simulink model "TAL8"  (Simulink 6.1)
settings: Solver=ode45  StartTime=0.0  StopTime=1000.0  RelTol=1e-3
values from neighbouring files (symbols this model uses):
  apr = 4    [data_TAL.m]
  apt = .3    (= 0.3)    [data_TAL.m]
  c_tal = 1    [data_TAL.m]
  egpith = -85    [data_synapses.m]
  ek_tal = -90    [data_TAL.m]
  el_tal = -70    [data_TAL.m]
  ena_tal = 50    [data_TAL.m]
  et_tal = 0    [data_TAL.m]
  ggpith = ggpith*mod_gpital    [CN_launch_CN_analyze_TAL2.m]    (also in CN_launch_sysTAL.m = ggpith*2; data_synapses.m = 0.06)
  gk_tal = 5    [data_TAL.m]
  gl_tal = 0.05    [data_TAL.m]
  gna_tal = 3    [data_TAL.m]
  gt_tal = 5    [data_TAL.m]
  ht0 = [i_v_16(322),i_v_16(325),i_v_16(322),i_v_16(325),i_v_16(322),i_v_16(325)]    [CN_launch_CN_analyze_TAL2.m]    (also in CN_launch_sysTAL.m)
  qht = 5.5    [data_TAL.m]
  rt0 = [i_v_16(323),i_v_16(326),i_v_16(323),i_v_16(326),i_v_16(323),i_v_16(326)]    [CN_launch_CN_analyze_TAL2.m]    (also in CN_launch_sysTAL.m)
  tadj = 1    [data_TAL.m]
  vt0 = [i_v_16(321),i_v_16(324),i_v_16(321),i_v_16(324),i_v_16(321),i_v_16(324)]    [CN_launch_CN_analyze_TAL2.m]    (also in CN_launch_sysTAL.m)
settings Model: LastModifiedBy=marco
settings DataIOCC: ExternalInput=[t2, u2]  LoadExternalInput=on
settings OptimizationCC: InlineInvariantSignals=off
settings DebuggingCC: SolverPrmCheckMsg=warning

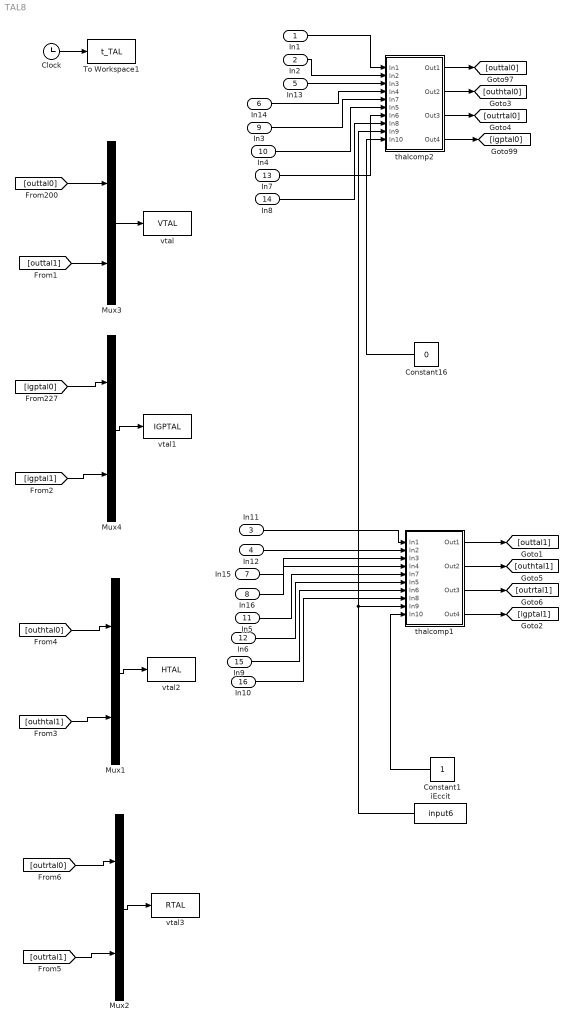
== system TAL8 ==
  In1 : Inport  Port=1  LatchInput=off
  In2 : Inport  Port=2  LatchInput=off
  In11 : Inport  Port=3  LatchInput=off
  In12 : Inport  Port=4  LatchInput=off
  In13 : Inport  Port=5  LatchInput=off
  In14 : Inport  Port=6  LatchInput=off
  In15 : Inport  Port=7  LatchInput=off
  In16 : Inport  Port=8  LatchInput=off
  In3 : Inport  Port=9  LatchInput=off
  In4 : Inport  Port=10  LatchInput=off
  In5 : Inport  Port=11  LatchInput=off
  In6 : Inport  Port=12  LatchInput=off
  In7 : Inport  Port=13  LatchInput=off
  In8 : Inport  Port=14  LatchInput=off
  In9 : Inport  Port=15  LatchInput=off
  In10 : Inport  Port=16  LatchInput=off
  Clock : Clock
      settings: Decimation=10
  Constant1 : Constant  Orientation=left
  Constant16 : Constant  Orientation=left  Value=0
  Mux{1..4} (4 alike) : Mux  Inputs=2
  To Workspace1 : ToWorkspace  VariableName=t_TAL  SampleTime=-1  SaveFormat=Array
  iEccit : FromWorkspace  Orientation=left  VariableName=input6  SampleTime=1
  thalcomp1 : Subsystem
  thalcomp2 : Subsystem
  vtal : ToWorkspace  VariableName=VTAL  SampleTime=-1  SaveFormat=Array
  vtal1 : ToWorkspace  VariableName=IGPTAL  SampleTime=-1  SaveFormat=Array
  vtal2 : ToWorkspace  VariableName=HTAL  SampleTime=-1  SaveFormat=Array
  vtal3 : ToWorkspace  VariableName=RTAL  SampleTime=-1  SaveFormat=Array
  wires:
  Clock/1 -> To Workspace1/1
  thalcomp2/1(Out1) -> [outtal0]
  In2/1 -> thalcomp2/2(In2)
  thalcomp2/4(Out4) -> [igptal0]
  In1/1 -> thalcomp2/1(In1)
  Mux3/1 -> vtal/1
  [outtal0] -> Mux3/1
  Mux4/1 -> vtal1/1
  [igptal0] -> Mux4/1
  In13/1 -> thalcomp2/3(In3)
  In14/1 -> thalcomp2/4(In4)
  Constant16/1 -> thalcomp2/10(In10)
  iEccit/1 -> thalcomp2/9(In9), thalcomp1/9(In9)
  In3/1 -> thalcomp2/5(In7)
  In4/1 -> thalcomp2/6(In5)
  In7/1 -> thalcomp2/7(In6)
  In8/1 -> thalcomp2/8(In8)
  Constant1/1 -> thalcomp1/10(In10)
  In11/1 -> thalcomp1/1(In1)
  In12/1 -> thalcomp1/2(In2)
  In15/1 -> thalcomp1/3(In3)
  In16/1 -> thalcomp1/4(In4)
  In5/1 -> thalcomp1/5(In7)
  In6/1 -> thalcomp1/6(In5)
  In9/1 -> thalcomp1/7(In6)
  In10/1 -> thalcomp1/8(In8)
  thalcomp1/1(Out1) -> [outtal1]
  thalcomp1/4(Out4) -> [igptal1]
  [outtal1] -> Mux3/2
  [igptal1] -> Mux4/2
  thalcomp2/2(Out2) -> [outhtal0]
  thalcomp2/3(Out3) -> [outrtal0]
  thalcomp1/2(Out2) -> [outhtal1]
  thalcomp1/3(Out3) -> [outrtal1]
  Mux1/1 -> vtal2/1
  [outhtal0] -> Mux1/1
  [outhtal1] -> Mux1/2
  Mux2/1 -> vtal3/1
  [outrtal0] -> Mux2/1
  [outrtal1] -> Mux2/2

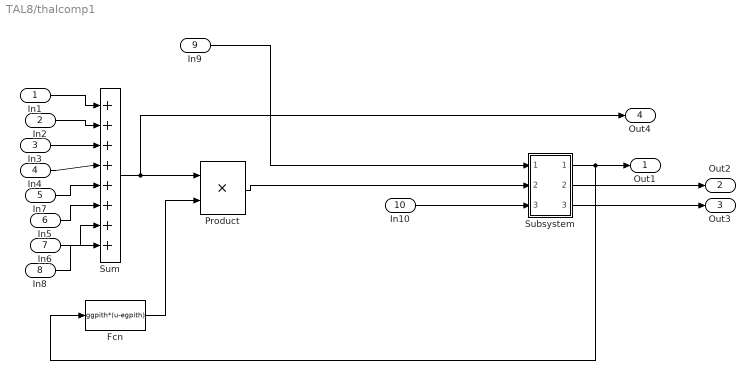
== system TAL8/thalcomp1 ==
  In1 : Inport  Port=1  LatchInput=off
  In2 : Inport  Port=2  LatchInput=off
  In3 : Inport  Port=3  LatchInput=off
  In4 : Inport  Port=4  LatchInput=off
  In7 : Inport  Port=5  LatchInput=off
  In5 : Inport  Port=6  LatchInput=off
  In6 : Inport  Port=7  LatchInput=off
  In8 : Inport  Port=8  LatchInput=off
  In9 : Inport  Port=9  LatchInput=off
  In10 : Inport  Port=10  LatchInput=off
  Fcn : Fcn  Expr=ggpith*(u-egpith)
  Product : Product  SaturateOnIntegerOverflow=on  InputSameDT=on
  Subsystem : Subsystem
  Sum : Sum  Inputs=++++++++  SaturateOnIntegerOverflow=on  InputSameDT=on
  Out1 : Outport
  Out2 : Outport  Port=2
  Out3 : Outport  Port=3
  Out4 : Outport  Port=4
  wires:
  Sum/1 -> Product/1, Out4/1
  Fcn/1 -> Product/2
  In1/1 -> Sum/1
  In2/1 -> Sum/2
  Product/1 -> Subsystem/2(In2)
  In9/1 -> Subsystem/1(In1)
  Subsystem/1(Out1) -> Fcn/1, Out1/1
  In10/1 -> Subsystem/3(In3)
  In4/1 -> Sum/4
  In3/1 -> Sum/3
  In8/1 -> Sum/8
  In6/1 -> Sum/7
  In5/1 -> Sum/6
  In7/1 -> Sum/5
  Subsystem/2(Out2) -> Out2/1
  Subsystem/3(Out3) -> Out3/1

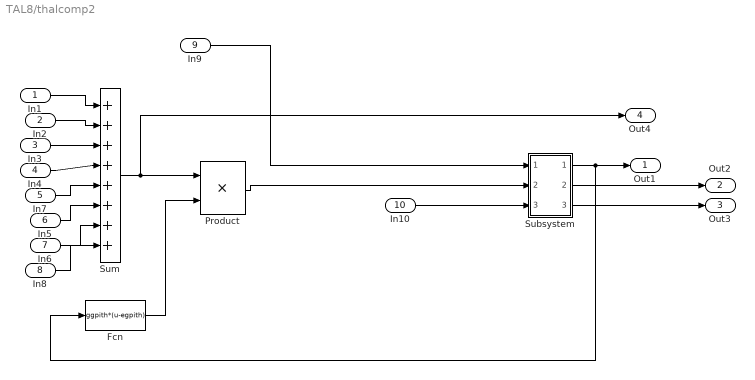
== system TAL8/thalcomp2 ==
  In1 : Inport  Port=1  LatchInput=off
  In2 : Inport  Port=2  LatchInput=off
  In3 : Inport  Port=3  LatchInput=off
  In4 : Inport  Port=4  LatchInput=off
  In7 : Inport  Port=5  LatchInput=off
  In5 : Inport  Port=6  LatchInput=off
  In6 : Inport  Port=7  LatchInput=off
  In8 : Inport  Port=8  LatchInput=off
  In9 : Inport  Port=9  LatchInput=off
  In10 : Inport  Port=10  LatchInput=off
  Fcn : Fcn  Expr=ggpith*(u-egpith)
  Product : Product  SaturateOnIntegerOverflow=on  InputSameDT=on
  Subsystem : Subsystem
  Sum : Sum  Inputs=++++++++  SaturateOnIntegerOverflow=on  InputSameDT=on
  Out1 : Outport
  Out2 : Outport  Port=2
  Out3 : Outport  Port=3
  Out4 : Outport  Port=4
  wires:
  Sum/1 -> Product/1, Out4/1
  Fcn/1 -> Product/2
  In1/1 -> Sum/1
  In2/1 -> Sum/2
  Product/1 -> Subsystem/2(In2)
  In9/1 -> Subsystem/1(In1)
  Subsystem/1(Out1) -> Fcn/1, Out1/1
  In10/1 -> Subsystem/3(In3)
  In4/1 -> Sum/4
  In3/1 -> Sum/3
  In8/1 -> Sum/8
  In6/1 -> Sum/7
  In5/1 -> Sum/6
  In7/1 -> Sum/5
  Subsystem/2(Out2) -> Out2/1
  Subsystem/3(Out3) -> Out3/1

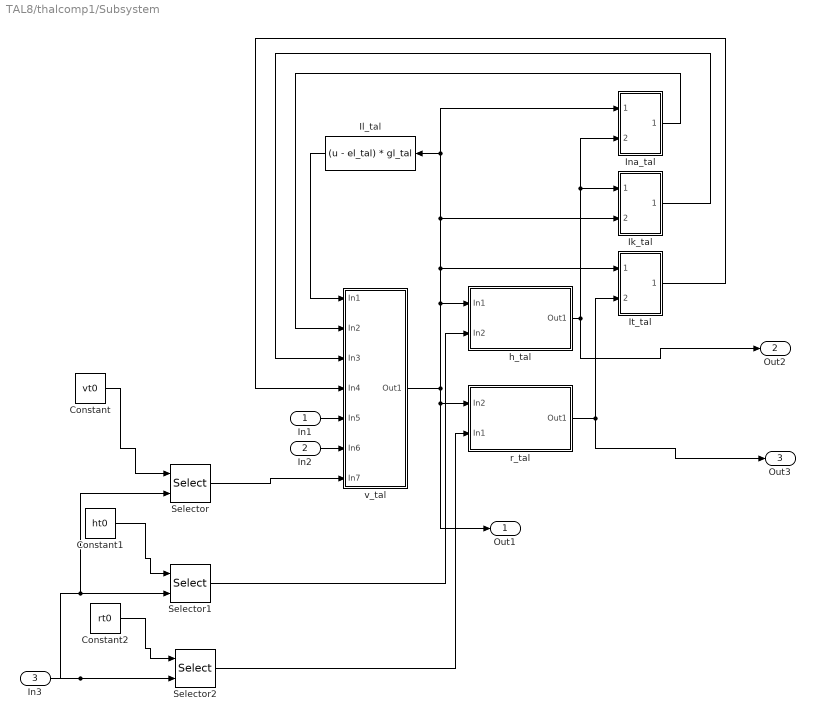
== system TAL8/thalcomp1/Subsystem ==
  In1 : Inport  Port=1  LatchInput=off
  In2 : Inport  Port=2  LatchInput=off
  In3 : Inport  Port=3  LatchInput=off
  Constant : Constant  Value=vt0
  Constant1 : Constant  Value=ht0
  Constant2 : Constant  Value=rt0
  Ik_tal : Subsystem
  Il_tal : Fcn  Orientation=left  Expr=(u - el_tal) * gl_tal
  Ina_tal : Subsystem
  It_tal : Subsystem
  Selector : Selector  IndexMode=Zero-based  ElementSrc=External  Elements=[1 3]
  Selector1 : Selector  IndexMode=Zero-based  ElementSrc=External  Elements=[1 3]
  Selector2 : Selector  IndexMode=Zero-based  ElementSrc=External  Elements=[1 3]
  h_tal : Subsystem
  r_tal : Subsystem
  v_tal : Subsystem
  Out1 : Outport
  Out2 : Outport  Port=2
  Out3 : Outport  Port=3
  wires:
  Il_tal/1 -> v_tal/1(In1)
  Ina_tal/1(Out1) -> v_tal/2(In2)
  Ik_tal/1(Out1) -> v_tal/3(In3)
  h_tal/1(Out1) -> Ik_tal/1(In1), Ina_tal/2(In2), Out2/1
  r_tal/1(Out1) -> It_tal/2(In2), Out3/1
  It_tal/1(Out1) -> v_tal/4(In4)
  v_tal/1(Out1) -> Il_tal/1, Ina_tal/1(In1), Ik_tal/2(In2), It_tal/1(In1), h_tal/1(In1), r_tal/1(In2), Out1/1
  In1/1 -> v_tal/5(In5)
  In2/1 -> v_tal/6(In6)
  In3/1 -> Selector2/2, Selector1/2, Selector/2
  Constant/1 -> Selector/1
  Selector/1 -> v_tal/7(In7)
  Constant1/1 -> Selector1/1
  Selector1/1 -> h_tal/2(In2)
  Constant2/1 -> Selector2/1
  Selector2/1 -> r_tal/2(In1)

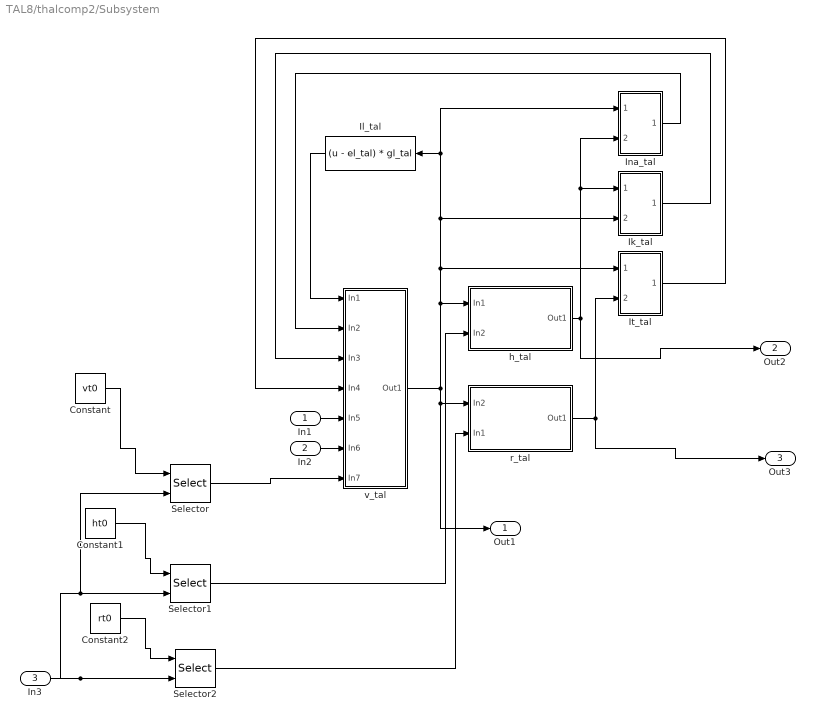
== system TAL8/thalcomp2/Subsystem ==
  In1 : Inport  Port=1  LatchInput=off
  In2 : Inport  Port=2  LatchInput=off
  In3 : Inport  Port=3  LatchInput=off
  Constant : Constant  Value=vt0
  Constant1 : Constant  Value=ht0
  Constant2 : Constant  Value=rt0
  Ik_tal : Subsystem
  Il_tal : Fcn  Orientation=left  Expr=(u - el_tal) * gl_tal
  Ina_tal : Subsystem
  It_tal : Subsystem
  Selector : Selector  IndexMode=Zero-based  ElementSrc=External  Elements=[1 3]
  Selector1 : Selector  IndexMode=Zero-based  ElementSrc=External  Elements=[1 3]
  Selector2 : Selector  IndexMode=Zero-based  ElementSrc=External  Elements=[1 3]
  h_tal : Subsystem
  r_tal : Subsystem
  v_tal : Subsystem
  Out1 : Outport
  Out2 : Outport  Port=2
  Out3 : Outport  Port=3
  wires:
  Il_tal/1 -> v_tal/1(In1)
  Ina_tal/1(Out1) -> v_tal/2(In2)
  Ik_tal/1(Out1) -> v_tal/3(In3)
  h_tal/1(Out1) -> Ik_tal/1(In1), Ina_tal/2(In2), Out2/1
  r_tal/1(Out1) -> It_tal/2(In2), Out3/1
  It_tal/1(Out1) -> v_tal/4(In4)
  v_tal/1(Out1) -> Il_tal/1, Ina_tal/1(In1), Ik_tal/2(In2), It_tal/1(In1), h_tal/1(In1), r_tal/1(In2), Out1/1
  In1/1 -> v_tal/5(In5)
  In2/1 -> v_tal/6(In6)
  In3/1 -> Selector2/2, Selector1/2, Selector/2
  Constant/1 -> Selector/1
  Selector/1 -> v_tal/7(In7)
  Constant1/1 -> Selector1/1
  Selector1/1 -> h_tal/2(In2)
  Constant2/1 -> Selector2/1
  Selector2/1 -> r_tal/2(In1)

== system TAL8/thalcomp1/Subsystem/Ik_tal ==
  In1 : Inport  Port=1  LatchInput=off
  In2 : Inport  Port=2  LatchInput=off
  Fcn : Fcn  Expr=gk_tal * ((0.75 * (1-u)) ^ 4)
  Fcn1 : Fcn  Expr=u - ek_tal
  Product : Product  SaturateOnIntegerOverflow=on  InputSameDT=on
  Out1 : Outport
  wires:
  Fcn/1 -> Product/1
  Fcn1/1 -> Product/2
  In1/1 -> Fcn/1
  In2/1 -> Fcn1/1
  Product/1 -> Out1/1

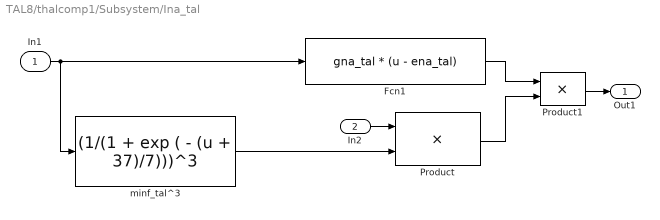
== system TAL8/thalcomp1/Subsystem/Ina_tal ==
  In1 : Inport  Port=1  LatchInput=off
  In2 : Inport  Port=2  LatchInput=off
  Fcn1 : Fcn  Expr=gna_tal * (u - ena_tal)
  Product : Product  SaturateOnIntegerOverflow=on  InputSameDT=on
  Product1 : Product  SaturateOnIntegerOverflow=on  InputSameDT=on
  minf_tal^3 : Fcn  Expr=(1/(1 + exp ( - (u + 37)/7)))^3
  Out1 : Outport
  wires:
  minf_tal^3/1 -> Product/2
  Product/1 -> Product1/2
  Fcn1/1 -> Product1/1
  In2/1 -> Product/1
  Product1/1 -> Out1/1
  In1/1 -> minf_tal^3/1, Fcn1/1

== system TAL8/thalcomp1/Subsystem/It_tal ==
  In1 : Inport  Port=1  LatchInput=off
  In2 : Inport  Port=2  LatchInput=off
  Fcn : Fcn  Expr=gt_tal * (u - et_tal)
  Product : Product  Inputs=3  SaturateOnIntegerOverflow=on  InputSameDT=on
  pinf_tal ^ 2 : Fcn  Expr=(1 / (1 + exp ( - (u + 60) / 6.2)))^2
  Out1 : Outport
  wires:
  In1/1 -> Fcn/1, pinf_tal ^ 2/1
  In2/1 -> Product/3
  pinf_tal ^ 2/1 -> Product/2
  Fcn/1 -> Product/1
  Product/1 -> Out1/1

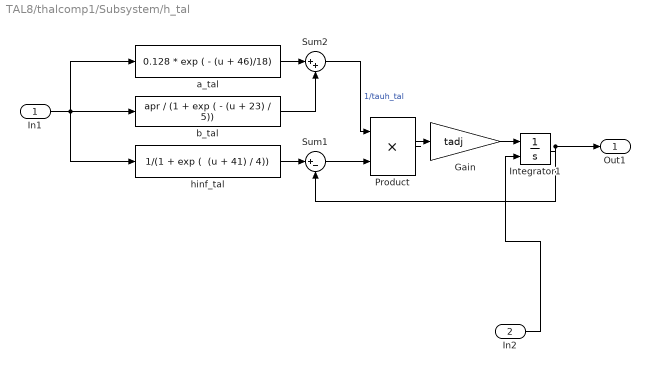
== system TAL8/thalcomp1/Subsystem/h_tal ==
  In1 : Inport  Port=1  LatchInput=off
  In2 : Inport  Port=2  LatchInput=off
  Gain : Gain  Gain=tadj
  Integrator1 : Integrator  InitialConditionSource=external
  Product : Product  SaturateOnIntegerOverflow=on  InputSameDT=on
  Sum1 : Sum  Inputs=|+-  SaturateOnIntegerOverflow=on  InputSameDT=on
  Sum2 : Sum  Inputs=|++  SaturateOnIntegerOverflow=on  InputSameDT=on
  a_tal : Fcn  Expr=0.128 * exp ( - (u + 46)/18)
  b_tal : Fcn  Expr=apr / (1 + exp ( - (u + 23) / 5))
  hinf_tal : Fcn  Expr="1/(1 + exp (  (u + 41) / 4))"
  Out1 : Outport
  wires:
  In1/1 -> a_tal/1, hinf_tal/1, b_tal/1
  a_tal/1 -> Sum2/1
  b_tal/1 -> Sum2/2
  Sum2/1 -> Product/1  "1/tauh_tal"
  Integrator1/1 -> Sum1/2, Out1/1
  hinf_tal/1 -> Sum1/1
  Sum1/1 -> Product/2
  In2/1 -> Integrator1/2
  Product/1 -> Gain/1
  Gain/1 -> Integrator1/1

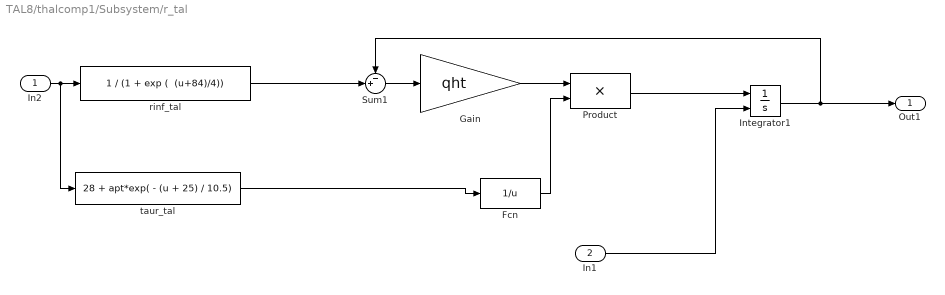
== system TAL8/thalcomp1/Subsystem/r_tal ==
  In2 : Inport  Port=1  LatchInput=off
  In1 : Inport  Port=2  LatchInput=off
  Fcn : Fcn  Expr=1/u
  Gain : Gain  Gain=qht
  Integrator1 : Integrator  InitialConditionSource=external
  Product : Product  SaturateOnIntegerOverflow=on  InputSameDT=on
  Sum1 : Sum  Inputs=-+|  SaturateOnIntegerOverflow=on  InputSameDT=on
  rinf_tal : Fcn  Expr="1 / (1 + exp (  (u+84)/4))"
  taur_tal : Fcn  Expr=28 + apt*exp( - (u + 25) / 10.5)
  Out1 : Outport
  wires:
  rinf_tal/1 -> Sum1/2
  taur_tal/1 -> Fcn/1
  Fcn/1 -> Product/2
  Product/1 -> Integrator1/1
  Integrator1/1 -> Out1/1, Sum1/1
  In2/1 -> rinf_tal/1, taur_tal/1
  In1/1 -> Integrator1/2
  Sum1/1 -> Gain/1
  Gain/1 -> Product/1

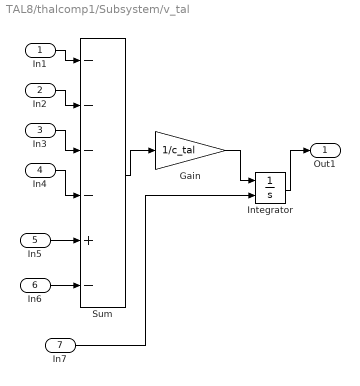
== system TAL8/thalcomp1/Subsystem/v_tal ==
  In1 : Inport  Port=1  LatchInput=off
  In2 : Inport  Port=2  LatchInput=off
  In3 : Inport  Port=3  LatchInput=off
  In4 : Inport  Port=4  LatchInput=off
  In5 : Inport  Port=5  LatchInput=off
  In6 : Inport  Port=6  LatchInput=off
  In7 : Inport  Port=7  LatchInput=off
  Gain : Gain  Gain=1/c_tal  SaturateOnIntegerOverflow=on
  Integrator : Integrator  InitialConditionSource=external  InitialCondition=-80  LimitOutput=on  UpperSaturationLimit=80
  Sum : Sum  Inputs=----+-  SaturateOnIntegerOverflow=on  InputSameDT=on
  Out1 : Outport
  wires:
  Sum/1 -> Gain/1
  Gain/1 -> Integrator/1
  In1/1 -> Sum/1
  In2/1 -> Sum/2
  In3/1 -> Sum/3
  Integrator/1 -> Out1/1
  In4/1 -> Sum/4
  In5/1 -> Sum/5
  In6/1 -> Sum/6
  In7/1 -> Integrator/2

== system TAL8/thalcomp2/Subsystem/Ik_tal ==
  In1 : Inport  Port=1  LatchInput=off
  In2 : Inport  Port=2  LatchInput=off
  Fcn : Fcn  Expr=gk_tal * ((0.75 * (1-u)) ^ 4)
  Fcn1 : Fcn  Expr=u - ek_tal
  Product : Product  SaturateOnIntegerOverflow=on  InputSameDT=on
  Out1 : Outport
  wires:
  Fcn/1 -> Product/1
  Fcn1/1 -> Product/2
  In1/1 -> Fcn/1
  In2/1 -> Fcn1/1
  Product/1 -> Out1/1

== system TAL8/thalcomp2/Subsystem/Ina_tal ==
  In1 : Inport  Port=1  LatchInput=off
  In2 : Inport  Port=2  LatchInput=off
  Fcn1 : Fcn  Expr=gna_tal * (u - ena_tal)
  Product : Product  SaturateOnIntegerOverflow=on  InputSameDT=on
  Product1 : Product  SaturateOnIntegerOverflow=on  InputSameDT=on
  minf_tal^3 : Fcn  Expr=(1/(1 + exp ( - (u + 37)/7)))^3
  Out1 : Outport
  wires:
  minf_tal^3/1 -> Product/2
  Product/1 -> Product1/2
  Fcn1/1 -> Product1/1
  In2/1 -> Product/1
  Product1/1 -> Out1/1
  In1/1 -> minf_tal^3/1, Fcn1/1

== system TAL8/thalcomp2/Subsystem/It_tal ==
  In1 : Inport  Port=1  LatchInput=off
  In2 : Inport  Port=2  LatchInput=off
  Fcn : Fcn  Expr=gt_tal * (u - et_tal)
  Product : Product  Inputs=3  SaturateOnIntegerOverflow=on  InputSameDT=on
  pinf_tal ^ 2 : Fcn  Expr=(1 / (1 + exp ( - (u + 60) / 6.2)))^2
  Out1 : Outport
  wires:
  In1/1 -> Fcn/1, pinf_tal ^ 2/1
  In2/1 -> Product/3
  pinf_tal ^ 2/1 -> Product/2
  Fcn/1 -> Product/1
  Product/1 -> Out1/1

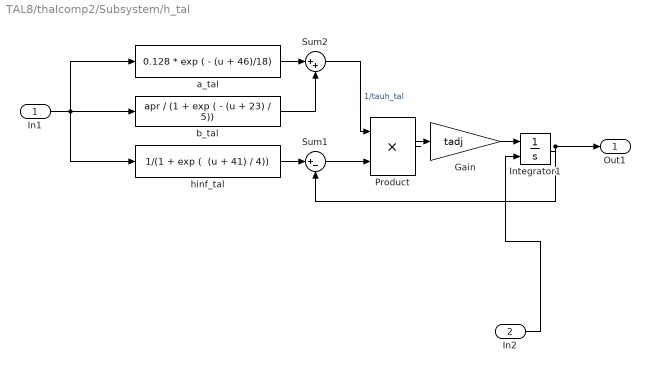
== system TAL8/thalcomp2/Subsystem/h_tal ==
  In1 : Inport  Port=1  LatchInput=off
  In2 : Inport  Port=2  LatchInput=off
  Gain : Gain  Gain=tadj
  Integrator1 : Integrator  InitialConditionSource=external
  Product : Product  SaturateOnIntegerOverflow=on  InputSameDT=on
  Sum1 : Sum  Inputs=|+-  SaturateOnIntegerOverflow=on  InputSameDT=on
  Sum2 : Sum  Inputs=|++  SaturateOnIntegerOverflow=on  InputSameDT=on
  a_tal : Fcn  Expr=0.128 * exp ( - (u + 46)/18)
  b_tal : Fcn  Expr=apr / (1 + exp ( - (u + 23) / 5))
  hinf_tal : Fcn  Expr="1/(1 + exp (  (u + 41) / 4))"
  Out1 : Outport
  wires:
  In1/1 -> a_tal/1, hinf_tal/1, b_tal/1
  a_tal/1 -> Sum2/1
  b_tal/1 -> Sum2/2
  Sum2/1 -> Product/1  "1/tauh_tal"
  Integrator1/1 -> Sum1/2, Out1/1
  hinf_tal/1 -> Sum1/1
  Sum1/1 -> Product/2
  In2/1 -> Integrator1/2
  Product/1 -> Gain/1
  Gain/1 -> Integrator1/1

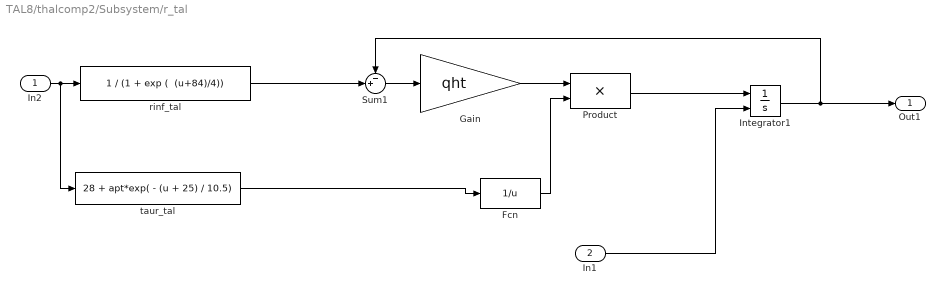
== system TAL8/thalcomp2/Subsystem/r_tal ==
  In2 : Inport  Port=1  LatchInput=off
  In1 : Inport  Port=2  LatchInput=off
  Fcn : Fcn  Expr=1/u
  Gain : Gain  Gain=qht
  Integrator1 : Integrator  InitialConditionSource=external
  Product : Product  SaturateOnIntegerOverflow=on  InputSameDT=on
  Sum1 : Sum  Inputs=-+|  SaturateOnIntegerOverflow=on  InputSameDT=on
  rinf_tal : Fcn  Expr="1 / (1 + exp (  (u+84)/4))"
  taur_tal : Fcn  Expr=28 + apt*exp( - (u + 25) / 10.5)
  Out1 : Outport
  wires:
  rinf_tal/1 -> Sum1/2
  taur_tal/1 -> Fcn/1
  Fcn/1 -> Product/2
  Product/1 -> Integrator1/1
  Integrator1/1 -> Out1/1, Sum1/1
  In2/1 -> rinf_tal/1, taur_tal/1
  In1/1 -> Integrator1/2
  Sum1/1 -> Gain/1
  Gain/1 -> Product/1

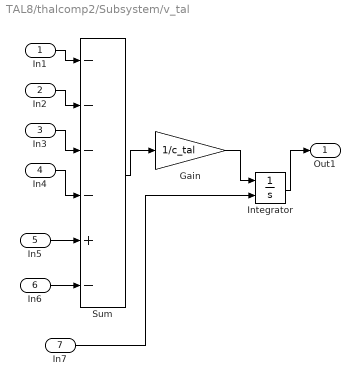
== system TAL8/thalcomp2/Subsystem/v_tal ==
  In1 : Inport  Port=1  LatchInput=off
  In2 : Inport  Port=2  LatchInput=off
  In3 : Inport  Port=3  LatchInput=off
  In4 : Inport  Port=4  LatchInput=off
  In5 : Inport  Port=5  LatchInput=off
  In6 : Inport  Port=6  LatchInput=off
  In7 : Inport  Port=7  LatchInput=off
  Gain : Gain  Gain=1/c_tal  SaturateOnIntegerOverflow=on
  Integrator : Integrator  InitialConditionSource=external  InitialCondition=-80  LimitOutput=on  UpperSaturationLimit=80
  Sum : Sum  Inputs=----+-  SaturateOnIntegerOverflow=on  InputSameDT=on
  Out1 : Outport
  wires:
  Sum/1 -> Gain/1
  Gain/1 -> Integrator/1
  In1/1 -> Sum/1
  In2/1 -> Sum/2
  In3/1 -> Sum/3
  Integrator/1 -> Out1/1
  In4/1 -> Sum/4
  In5/1 -> Sum/5
  In6/1 -> Sum/6
  In7/1 -> Integrator/2
